simulink library "DQ_SR_LIB_SIM"  (R2019b)
settings: Solver=VariableStepAuto  StartTime=0.0  StopTime=10.0  RelTol=1e-3  EnableMultiTasking=on
undefined symbols (not defined in the file): crossqm, II, II0, magnitude, SATFUNCNAME, X0, XCG0, xi0
(part 1 of 2)
settings Model: Creator=rivolta  LastModifiedBy=AurelianoRivolta
settings DataIOCC: LimitDataPoints=on  ReturnWorkspaceOutputs=off
settings OptimizationCC: LifeSpan=inf
settings DebuggingCC: AllowSymbolicDim=off  SFUnexpectedBacktrackingDiag=warning  SFNoUnconditionalDefaultTransitionDiag=warning  SFExecutionAtInitializationDiag=none  ArithmeticOperatorsInVariantConditions=warning
settings ModelReferenceCC: PropagateSignalLabelsOutOfModel=off
settings SFSimCC: SimUseLocalCustomCode=off  CustomCodeUndefinedFunction=UseInterfaceOnly
settings RTWCC: RTWUseLocalCustomCode=off
settings CodeAppCC: StateflowObjectComments=on
settings GRTTargetCC: TargetLangStandard=C89/C90 (ANSI)
settings ConfigComp: CovMetricSettings=dw  CovHtmlReporting=on  CovSaveCumulativeToWorkspaceVar=on  CovSaveSingleToWorkspaceVar=on  CovExternalEMLEnable=off

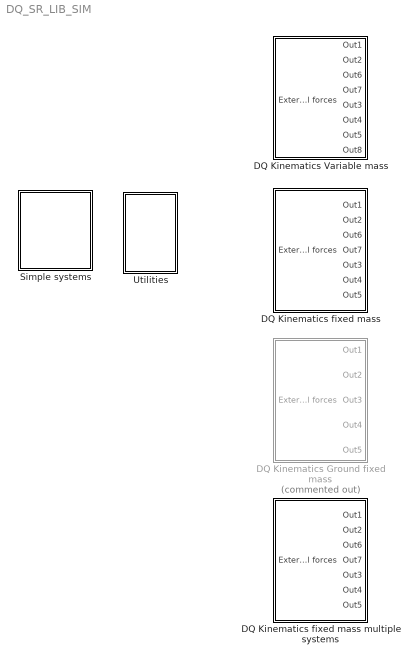
== system DQ_SR_LIB_SIM ==
  DQ Kinematics Ground fixed mass : Subsystem  Commented=on  mask{dynfun=SATFUNCNAME, Gswitch=ECI gravity (F,T), n_bodies=2, n_var0=5, n_ext=7, q_norm_in=[6:9;1:4], II=II, X0=X0, UPPERSAT=Inf, LOWERSAT=-Inf}
      mask prompts: dynfun "System function"; Gswitch "Gravity model"; n_bodies "Number of bodies"; n_var0 "Number of variables"; n_ext "External force size"; q_norm_in "Quaternion indeces"; II "Mass matrix"; X0 "System"; UPPERSAT "Upper Limit"; LOWERSAT "Lower Limit"
      mask init:
      | % check if the incoming function has the correct number of inputs
      | if nargin(dynfun) ~= 9
      |     error('wrong number of inputs, should be: [x,dx,xcg,vcg,time,II,ext_forces,xi]')
      | end
      | 
      | % number of state variables as from input
      | n_var0=length(X0)/2;
      | 
      | % number of bodies from mass conditions
      | n_bodies=size(II,2);
      | 
      | % convert function to be used for trials
      | trialf=str2func(dynfun);
      | gfun=str2func('NO_gravity');
      | 
      | % supposed length of external forces vector
      | n_ext=1;
      | 
      | % check variables
      | CKH=true;
      | iter = 0;
      | line_err=1e5;
      | xi0=0;
      | 
      | while CKH && iter<100
      | 
      |     try 
      |         trialf(ones(n_var0,1),ones(n_var0,1),ones(3,1),ones(3,1),0,II,ones(n_ext,1),xi0,gfun);
      |         CKH=false;
      |     catch M
      |         % catch error line
      |         G=M.stack.line;
      |         % check if the error is after previous line
      |         if (G <= line_err)
      |             n_ext=n_ext+1;
      |         end
      |         % adjourne line error
      |         line_err=G;
      |     end
      |     iter = iter +1;
      |     
      | end
      | 
      | % check if something went wrong. unlikely to have 100 input vector, to be
      | % fixed in later versions
      | if iter >100
      |     warning('likely to have inputs dimension incompatibility')
      | end
      | 
      | % check if I-O dimensions are consistent
      | sys=trialf(X0(n_var0+1:end),X0(1:n_var0),[],[],0,II,ones(n_ext,1),1,gfun);
      | 
      | if sys.n_bodies ~= n_bodies
      |     error('body number inconsistent')
      | end
      | 
      | if sys.nvar ~= n_var0
      |     error ('variable number inconsistent')
      | end
      | 
      | % convert to supply the function name to Mfunction
      | sys_gen_fun_NAME=uint8(dynfun);
      | 
      | % gravity function translation for Mfunction input
      | gravity_fun_NAME = select_gravity_model(Gswitch);
      | 
      | % state and its derivative size
      | n_var=2*n_var0;
      | 
      | % number of variable mass states
      | n_massvar=size(xi0);
      mask Help:
      | % Author: Aureliano Rivolta
      | % e-mail: aureliano.rivolta@polimi.it
      | % year: 2016
      | % private use only
      mask TypeOptions Gswitch: No gravity | Ground gravity (-z) | ECI gravity force | ECI gravity (F,T)
      mask DialogControl Container4 Prompt: System parameters
      mask DialogControl Container5 Prompt: Phisical parameters
      mask DialogControl Control3 Prompt: Initial conditions
      mask DialogControl Container3 Prompt: State Saturation
      mask DialogControl Control2 Prompt: Saturation limits for the system states. If no limits, then put Inf.
      mask Display:
      | port_label('input',1,'f_{ext}','interpreter','tex');
      | port_label('output',1,'v','interpreter','tex');
      | port_label('output',2,'x','interpreter','tex');
      | port_label('output',3,'a','interpreter','tex');
      | port_label('output',4,'da','interpreter','tex');
      | port_label('output',5,'dda','interpreter','tex');
      | fprintf('Ground\nfixed\nmass\nELIMINATO')
  DQ Kinematics Variable mass : Subsystem  mask{dynfun=SATFUNCNAME, Gswitch=No gravity, n_bodies=1, n_var0=4, n_ext=6, q_norm_in=[1:4]', NORMONOFF=on, II=II, xi0=xi0, X0=X0, XCG0=XCG0, UPPERSAT=Inf, LOWERSAT=-Inf}
      mask prompts: dynfun "System function"; Gswitch "Gravity model"; n_bodies "Number of bodies"; n_var0 "Number of variables"; n_ext "External force size"; q_norm_in "Quaternion indeces"; NORMONOFF "Normalize quaternions"; II "Mass matrix"; xi0 "Variable mass IC"; X0 "System"; XCG0 "Center of Mass"; UPPERSAT "Upper Limit"; LOWERSAT "Lower Limit"
      mask init:
      | % check if the incoming function has the correct number of inputs
      | if nargin(dynfun) ~= 9
      |     error('wrong number of inputs, should be: [x,dx,xcg,vcg,time,II,ext_forces,xi,gravity_fun]')
      | end
      | 
      | % number of state variables as from input
      | n_var0=length(X0)/2;
      | 
      | % number of bodies from mass conditions
      | n_bodies=size(II,2);
      | 
      | % convert function to be used for trials
      | trialf=str2func(dynfun);
      | gfun=str2func('NO_gravity');
      | 
      | % supposed length of external forces vector
      | n_ext=1;
      | 
      | % check variables
      | CKH=true;
      | iter = 0;
      | line_err=1e5;
      | 
      | while CKH && iter<100
      | 
      |     try 
      |         trialf(ones(n_var0,1),ones(n_var0,1),ones(3,1),ones(3,1),0,II,ones(n_ext,1),xi0,gfun);
      |         CKH=false;
      |     catch M
      |         % catch error line
      |         G=M.stack.line;
      |         % check if the error is after previous line
      |         if (G <= line_err)
      |             n_ext=n_ext+1;
      |         end
      |         % adjourne line error
      |         line_err=G;
      |     end
      |     iter = iter +1;
      |     
      | end
      | 
      | % check if something went wrong. unlikely to have 100 input vector, to be
      | % fixed in later versions
      | if iter >100
      |     warning('likely to have inputs dimension incompatibility')
      | end
      | 
      | % check if I-O dimensions are consistent
      | sys=trialf(X0(n_var0+1:end),X0(1:n_var0),XCG0(4:end),XCG0(1:3),0,II,ones(n_ext,1),xi0,gfun);
      | 
      | if sys.n_bodies ~= n_bodies
      |     error('body number inconsistent')
      | end
      | 
      | if sys.nvar ~= n_var0
      |     error ('variable number inconsistent')
      | end
      | 
      | % convert to supply the function name to Mfunction
      | sys_gen_fun_NAME=uint8(dynfun);
      | 
      | % gravity function translation for Mfunction input
      | gravity_fun_NAME = select_gravity_model(Gswitch);
      | 
      | % state and its derivative size
      | n_var=2*n_var0;
      | 
      | % number of variable mass states
      | n_massvar=size(xi0);
      mask Help:
      | % Author: Aureliano Rivolta
      | % e-mail: aureliano.rivolta@polimi.it
      | % year: 2016
      | % private use only
      mask TypeOptions Gswitch: No gravity | Ground gravity (-z) | ECI gravity force | ECI gravity (F,T) | CW linearized
      mask DialogControl Container4 Prompt: System parameters
      mask DialogControl Control5 Prompt: Edit
      mask DialogControl Control5 Callback:
      | fun2edit = eval(get_param(gcb,'dynfun'));
      | 
      | edit(fun2edit)
      mask DialogControl Control6 Prompt: New
      mask DialogControl Control6 Callback:
      | directory_string = get_DQ_folder;
      | 
      | copyfile([directory_string,'\simulink_blocks\onesat_S.m'],'template.m')
      | 
      | edit template
      mask DialogControl Container5 Prompt: Phisical parameters
      mask DialogControl Control3 Prompt: Initial conditions
      mask DialogControl Container3 Prompt: State Saturation
      mask DialogControl Control2 Prompt: Saturation limits for the system states. If no limits, then put Inf.
      mask Display:
      | port_label('input',1,'f_{ext}','interpreter','tex');
      | port_label('output',1,'v','interpreter','tex');
      | port_label('output',2,'x','interpreter','tex');
      | port_label('output',3,'v_{cg}','interpreter','tex');
      | port_label('output',4,'x_{cg}','interpreter','tex');
      | port_label('output',5,'a','interpreter','tex');
      | port_label('output',6,'da','interpreter','tex');
      | port_label('output',7,'dda','interpreter','tex');
      | port_label('output',8,'\xi','interpreter','tex');
      | fprintf('variable\nmass')
  DQ Kinematics fixed mass : Subsystem  mask{dynfun=SATFUNCNAME, Gswitch=No gravity, n_bodies=2, n_var0=5, n_ext=7, q_norm_in=[1:4]', NORMONOFF=on, II=II0, X0=X0, XCG0=XCG0, UPPERSAT=Inf, LOWERSAT=-Inf}
      mask prompts: dynfun "System function"; Gswitch "Gravity model:"; n_bodies "Number of bodies"; n_var0 "Number of variables"; n_ext "External force size"; q_norm_in "Quaternion indeces"; NORMONOFF "Normalize quaternion"; II "Mass matrix"; X0 "System"; XCG0 "Center of Mass"; UPPERSAT "Upper Limit"; LOWERSAT "Lower Limit"
      mask init:
      | % check if the incoming function has the correct number of inputs
      | if nargin(dynfun) ~= 9
      |     error('wrong number of inputs, should be: [x,dx,xcg,vcg,time,II,ext_forces,xi]')
      | end
      | 
      | % number of state variables as from input
      | n_var0=length(X0)/2;
      | 
      | % number of bodies from mass conditions
      | n_bodies=size(II,2);
      | 
      | % convert function to be used for trials
      | trialf=str2func(dynfun);
      | gfun=str2func('NO_gravity');
      | 
      | % supposed length of external forces vector
      | n_ext=1;
      | 
      | % check variables
      | CKH=true;
      | iter = 0;
      | line_err=1e5;
      | xi0=0;
      | 
      | 
      | while CKH && iter<100
      | 
      |     try 
      |         trialf(ones(n_var0,1),ones(n_var0,1),ones(3,1),ones(3,1),0,II,ones(n_ext,1),xi0,gfun);
      |         CKH=false;
      |     catch M
      |         % catch error line
      |         G=M.stack.line;
      |         % check if the error is after previous line
      |         if (G <= line_err)
      |             n_ext=n_ext+1;
      |         end
      |         % adjourne line error
      |         line_err=G;
      |     end
      |     iter = iter +1;
      |     
      | end
      | 
      | % check if something went wrong. unlikely to have 100 input vector, to be
      | % fixed in later versions
      | if iter >100
      |     warning('likely to have inputs dimension incompatibility')
      | end
      | 
      | % check if I-O dimensions are consistent
      | sys=trialf(X0(n_var0+1:end),X0(1:n_var0),XCG0(4:end),XCG0(1:3),0,II,ones(n_ext,1),1,gfun);
      | 
      | if sys.n_bodies ~= n_bodies
      |     error('body number inconsistent')
      | end
      | 
      | if sys.nvar ~= n_var0
      |     error ('variable number inconsistent')
      | end
      | 
      | % convert to supply the function name to Mfunction
      | sys_gen_fun_NAME=uint8(dynfun);
      | 
      | % gravity function translation for Mfunction input
      | gravity_fun_NAME = select_gravity_model(Gswitch);
      | 
      | % state and its derivative size
      | n_var=2*n_var0;
      | 
      | % number of variable mass states
      | n_massvar=size(xi0);
      mask Help:
      | % Author: Aureliano Rivolta
      | % e-mail: aureliano.rivolta@polimi.it
      | % year: 2016
      | % private use only
      mask TypeOptions Gswitch: No gravity | Ground gravity (-z) | ECI gravity force | ECI gravity (F,T) | CW linearized model
      mask DialogControl Container4 Prompt: System parameters
      mask DialogControl Control5 Prompt: Edit
      mask DialogControl Control5 Callback:
      | fun2edit = eval(get_param(gcb,'dynfun'));
      | 
      | edit(fun2edit);
      mask DialogControl Control6 Prompt: New
      mask DialogControl Control6 Callback: get_DQSR_template
      mask DialogControl Container5 Prompt: Phisical parameters
      mask DialogControl Control3 Prompt: Initial conditions
      mask DialogControl Container3 Prompt: State Saturation
      mask DialogControl Control2 Prompt: Saturation limits for the system states. If no limits, then put Inf.
      mask Display:
      | port_label('input',1,'f_{ext}','interpreter','tex');
      | port_label('output',1,'v','interpreter','tex');
      | port_label('output',2,'x','interpreter','tex');
      | port_label('output',3,'v_{cg}','interpreter','tex');
      | port_label('output',4,'x_{cg}','interpreter','tex');
      | port_label('output',5,'a','interpreter','tex');
      | port_label('output',6,'da','interpreter','tex');
      | port_label('output',7,'dda','interpreter','tex');
      | fprintf('fixed\nmass')
  DQ Kinematics fixed mass multiple systems : Subsystem  mask{dynfun=SATFUNCNAME, Gswitch=No gravity, n_bodies=2, n_var0=5, n_ext=7, q_norm_in=[1:4;5:8]', NORMONOFF=on, II=II0, X0=X0, XCG0=XCG0, UPPERSAT=Inf, LOWERSAT=-Inf}
      mask prompts: dynfun "System function"; Gswitch "Gravity model"; n_bodies "Number of bodies"; n_var0 "Number of variables"; n_ext "External force size"; q_norm_in "Quaternion indeces"; NORMONOFF "Normalize quaternion"; II "Mass matrix"; X0 "System"; XCG0 "Center of Mass"; UPPERSAT "Upper Limit"; LOWERSAT "Lower Limit"
      mask init:
      | % check if the incoming function has the correct number of inputs
      | if nargin(dynfun) ~= 9
      |     error('wrong number of inputs, should be: [x,dx,xcg,vcg,time,II,ext_forces,xi]')
      | end
      | 
      | % number of state variables as from input
      | n_var0=length(X0)/2;
      | 
      | % number of bodies from mass conditions
      | n_bodies=size(II,2);
      | 
      | % convert function to be used for trials
      | trialf=str2func(dynfun);
      | gfun=str2func('NO_gravity');
      | 
      | % supposed length of external forces vector
      | n_ext=1;
      | 
      | % check variables
      | CKH=true;
      | iter = 0;
      | line_err=1e5;
      | xi0=0;
      | 
      | while CKH && iter<100
      | 
      |     try 
      |         SSS=trialf(X0(n_var0+1:end),X0(1:n_var0),XCG0(4:6,:),XCG0(1:3,:),0,II,ones(n_ext,1),xi0,gfun);
      |         CKH=false;
      | %         SSS
      |     catch M
      |         % catch error line
      |         G=M.stack.line;
      |         % check if the error is after previous line
      |         if (G <= line_err)
      |             n_ext=n_ext+1;
      |         end
      |         % adjourne line error
      |         line_err=G;
      |     end
      |     iter = iter +1;
      |     
      | end
      | 
      | % check if something went wrong. unlikely to have 100 input vector, to be
      | % fixed in later versions
      | if iter >100
      |     warning('likely to have inputs dimension incompatibility')
      | end
      | 
      | % check if I-O dimensions are consistent
      | systems=trialf(X0(n_var0+1:end),X0(1:n_var0),XCG0(4:6,:),XCG0(1:3,:),0,II,ones(n_ext,1),1,gfun);
      | ns=length(systems);
      | 
      | %check bodies and variable numbers
      | [nb,nv]=deal(zeros(1,ns));
      | for i=1:ns
      |     nb(i)=systems(i).n_bodies;
      |     nv(i)=systems(i).nvar;
      | end
      | 
      | if sum(nb) ~= n_bodies
      |     error('body number inconsistent')
      | end
      | 
      | if sum(nv) ~= n_var0
      |     error ('variable number inconsistent')
      | end
      | 
      | % convert to supply the function name to Mfunction
      | sys_gen_fun_NAME=uint8(dynfun);
      | 
      | % gravity function translation for Mfunction input
      | gravity_fun_NAME = select_gravity_model(Gswitch);
      | 
      | % state and its derivative size
      | n_var=2*n_var0;
      | 
      | % number of variable mass states
      | n_massvar=size(xi0);
      | 
      | % initialize the contact memory matrix
      | nc=sum(sum(nb'*nb-diag(diag(nb'*nb))))/2;
      | vref0=zeros(6,nc);
      | 
      | % initialize the contact table
      | CONTACTABLE0=[];
      | 
      | for i=1:ns-1
      |     for k=1:nb(i)
      |         for j=i+1:ns
      |             for l=1:nb(j)
      |                 CONTACTABLE0=[CONTACTABLE0;[i,k,j,l]];
      |             end
      |         end
      |     end
      | end
      | 
      | % disable warnings. not the best options but in many cases there will be
      | % warnings for some parallel faces in the contact determination. In the
      | % future cases then 
      | warning off
      mask Help:
      | % Author: Aureliano Rivolta
      | % e-mail: aureliano.rivolta@polimi.it
      | % year: 2016
      | % private use only
      mask TypeOptions Gswitch: No gravity | Ground gravity (-z) | ECI gravity force | ECI gravity (F,T) | CW linearized model
      mask DialogControl Container4 Prompt: System parameters
      mask DialogControl Control5 Prompt: Edit
      mask DialogControl Control5 Callback:
      | fun2edit = eval(get_param(gcb,'dynfun'));
      | 
      | edit(fun2edit)
      mask DialogControl Control6 Prompt: New
      mask DialogControl Control6 Callback: get_DQSR_template
      mask DialogControl Container5 Prompt: Phisical parameters
      mask DialogControl Control3 Prompt: Initial conditions
      mask DialogControl Container3 Prompt: State Saturation
      mask DialogControl Control2 Prompt: Saturation limits for the system states. If no limits, then put Inf.
      mask Display:
      | port_label('input',1,'f_{ext}','interpreter','tex');
      | port_label('output',1,'v','interpreter','tex');
      | port_label('output',2,'x','interpreter','tex');
      | port_label('output',3,'v_{cg}','interpreter','tex');
      | port_label('output',4,'x_{cg}','interpreter','tex');
      | port_label('output',5,'a','interpreter','tex');
      | port_label('output',6,'da','interpreter','tex');
      | port_label('output',7,'dda','interpreter','tex');
      | fprintf('fixed\nmass\nsystems')
  Simple systems : Subsystem
      settings: OpenFcn=SAMPLE_systems
  Utilities : Subsystem

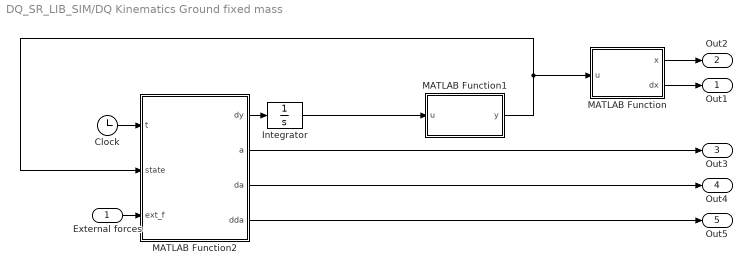
== system DQ_SR_LIB_SIM/DQ Kinematics Ground fixed mass ==
  External forces : Inport
  Clock : Clock
  Integrator : Integrator  InitialCondition=X0  LimitOutput=on  UpperSaturationLimit=UPPERSAT  LowerSaturationLimit=LOWERSAT
  MATLAB Function : MATLAB Function  TreatAsAtomicUnit=on  mask{n_states=n_var}
      mask prompts: n_states "Number of states"
  MATLAB Function1 : MATLAB Function  TreatAsAtomicUnit=on  mask{qindex=q_norm_in}
      mask prompts: qindex "Quaternion index"
      mask init:
      | index=qindex(1,:);
      | index2=qindex(2,:);
  MATLAB Function2 : MATLAB Function  TreatAsAtomicUnit=on
  Out1 : Outport
  Out2 : Outport  Port=2
  Out3 : Outport  Port=3
  Out4 : Outport  Port=4
  Out5 : Outport  Port=5
  wires:
  Clock/1 -> MATLAB Function2/1(t)
  MATLAB Function2/4(dda) -> Out5/1
  MATLAB Function/1(x) -> Out2/1
  MATLAB Function/2(dx) -> Out1/1
  MATLAB Function2/1(dy) -> Integrator/1
  MATLAB Function2/2(a) -> Out3/1
  MATLAB Function2/3(da) -> Out4/1
  External forces/1 -> MATLAB Function2/3(ext_f)
  Integrator/1 -> MATLAB Function1/1(u)
  MATLAB Function1/1(y) -> MATLAB Function/1(u), MATLAB Function2/2(state)

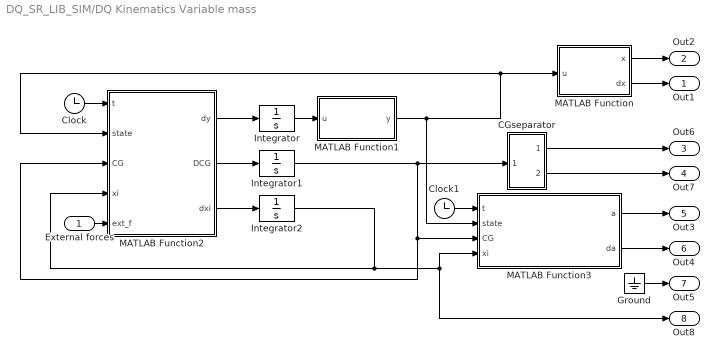
== system DQ_SR_LIB_SIM/DQ Kinematics Variable mass ==
  External forces : Inport
  CGseparator : Subsystem
      mask Display:
      | port_label('input',1,'CG')
      | port_label('output',1,'v_{cg}','interpreter','tex')
      | port_label('output',2,'x_{cg}','interpreter','tex')
  Clock : Clock
  Clock1 : Clock
  Ground : Ground
  Integrator : Integrator  InitialCondition=X0  LimitOutput=on  UpperSaturationLimit=UPPERSAT  LowerSaturationLimit=LOWERSAT
  Integrator1 : Integrator  InitialCondition=XCG0
  Integrator2 : Integrator  InitialCondition=xi0  LimitOutput=on  UpperSaturationLimit=1  LowerSaturationLimit=0
  MATLAB Function : MATLAB Function  TreatAsAtomicUnit=on  mask{n_states=n_var}
      mask prompts: n_states "Number of states"
  MATLAB Function1 : MATLAB Function  TreatAsAtomicUnit=on  mask{qindex=q_norm_in}
      mask prompts: qindex "Quaternion index"
  MATLAB Function2 : MATLAB Function  TreatAsAtomicUnit=on
  MATLAB Function3 : MATLAB Function  TreatAsAtomicUnit=on
  Out1 : Outport
  Out2 : Outport  Port=2
  Out6 : Outport  Port=3
  Out7 : Outport  Port=4
  Out3 : Outport  Port=5
  Out4 : Outport  Port=6
  Out5 : Outport  Port=7
  Out8 : Outport  Port=8
  wires:
  Integrator/1 -> MATLAB Function1/1(u)
  Integrator2/1 -> Out8/1, MATLAB Function3/4(xi), MATLAB Function2/4(xi)
  CGseparator/2(Out3) -> Out7/1
  External forces/1 -> MATLAB Function2/5(ext_f)
  MATLAB Function/2(dx) -> Out1/1
  MATLAB Function/1(x) -> Out2/1
  MATLAB Function2/2(DCG) -> Integrator1/1
  Clock/1 -> MATLAB Function2/1(t)
  CGseparator/1(Out1) -> Out6/1
  MATLAB Function2/3(dxi) -> Integrator2/1
  MATLAB Function1/1(y) -> MATLAB Function3/2(state), MATLAB Function2/2(state), MATLAB Function/1(u)
  MATLAB Function2/1(dy) -> Integrator/1
  Integrator1/1 -> CGseparator/1(In1), MATLAB Function2/3(CG), MATLAB Function3/3(CG)
  Clock1/1 -> MATLAB Function3/1(t)
  MATLAB Function3/1(a) -> Out3/1
  MATLAB Function3/2(da) -> Out4/1
  Ground/1 -> Out5/1

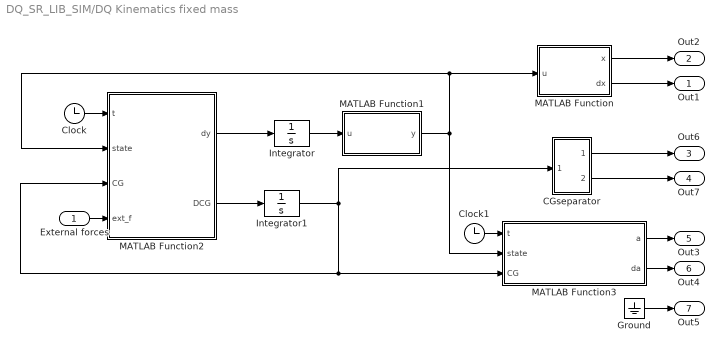
== system DQ_SR_LIB_SIM/DQ Kinematics fixed mass ==
  External forces : Inport
  CGseparator : Subsystem
      mask Display:
      | port_label('input',1,'CG')
      | port_label('output',1,'v_{cg}','interpreter','tex')
      | port_label('output',2,'x_{cg}','interpreter','tex')
  Clock : Clock
  Clock1 : Clock
  Ground : Ground
  Integrator : Integrator  InitialCondition=X0  LimitOutput=on  UpperSaturationLimit=UPPERSAT  LowerSaturationLimit=LOWERSAT
  Integrator1 : Integrator  InitialCondition=XCG0
  MATLAB Function : MATLAB Function  TreatAsAtomicUnit=on  mask{n_states=n_var}
      mask prompts: n_states "Number of states"
  MATLAB Function1 : MATLAB Function  TreatAsAtomicUnit=on  mask{qindex=q_norm_in}
      mask prompts: qindex "Quaternion index"
  MATLAB Function2 : MATLAB Function  TreatAsAtomicUnit=on
  MATLAB Function3 : MATLAB Function  TreatAsAtomicUnit=on
  Out1 : Outport
  Out2 : Outport  Port=2
  Out6 : Outport  Port=3
  Out7 : Outport  Port=4
  Out3 : Outport  Port=5
  Out4 : Outport  Port=6
  Out5 : Outport  Port=7
  wires:
  MATLAB Function1/1(y) -> MATLAB Function2/2(state), MATLAB Function/1(u), MATLAB Function3/2(state)
  CGseparator/2(Out3) -> Out7/1
  Integrator/1 -> MATLAB Function1/1(u)
  External forces/1 -> MATLAB Function2/4(ext_f)
  MATLAB Function2/1(dy) -> Integrator/1
  MATLAB Function/2(dx) -> Out1/1
  MATLAB Function/1(x) -> Out2/1
  MATLAB Function2/2(DCG) -> Integrator1/1
  Integrator1/1 -> CGseparator/1(In1), MATLAB Function3/3(CG), MATLAB Function2/3(CG)
  Clock/1 -> MATLAB Function2/1(t)
  CGseparator/1(Out1) -> Out6/1
  Clock1/1 -> MATLAB Function3/1(t)
  MATLAB Function3/1(a) -> Out3/1
  MATLAB Function3/2(da) -> Out4/1
  Ground/1 -> Out5/1

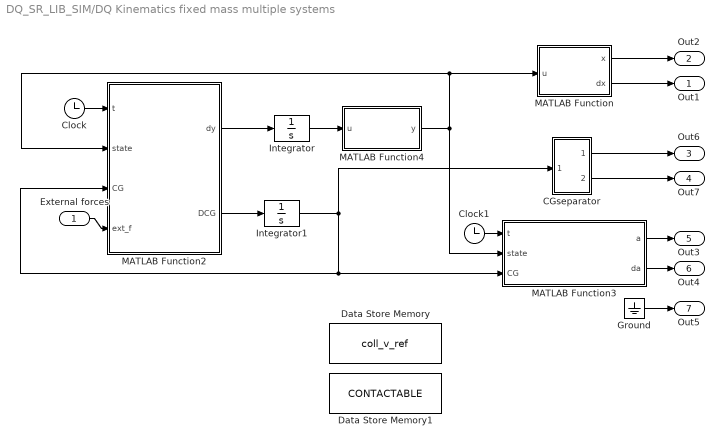
== system DQ_SR_LIB_SIM/DQ Kinematics fixed mass multiple systems ==
  External forces : Inport
  CGseparator : Subsystem
      mask Display:
      | port_label('input',1,'CG')
      | port_label('output',1,'v_{cg}','interpreter','tex')
      | port_label('output',2,'x_{cg}','interpreter','tex')
  Clock : Clock
  Clock1 : Clock
  Data Store Memory : DataStoreMemory  DataStoreName=coll_v_ref  ReadBeforeWriteMsg=warning  WriteAfterWriteMsg=warning  WriteAfterReadMsg=warning  InitialValue=vref0  VectorParams1D=off  ShowAdditionalParam=off  OutDataTypeStr=double  Dimensions=[6,nc]
  Data Store Memory1 : DataStoreMemory  DataStoreName=CONTACTABLE  ReadBeforeWriteMsg=warning  WriteAfterWriteMsg=warning  WriteAfterReadMsg=warning  InitialValue=CONTACTABLE0  VectorParams1D=off  ShowAdditionalParam=off  OutDataTypeStr=double  Dimensions=[nc,4]
  Ground : Ground
  Integrator : Integrator  InitialCondition=X0  LimitOutput=on  UpperSaturationLimit=UPPERSAT  LowerSaturationLimit=LOWERSAT
  Integrator1 : Integrator  InitialCondition=XCG0
  MATLAB Function : MATLAB Function  TreatAsAtomicUnit=on  mask{n_states=n_var}
      mask prompts: n_states "Number of states"
  MATLAB Function2 : MATLAB Function  TreatAsAtomicUnit=on
  MATLAB Function3 : MATLAB Function  TreatAsAtomicUnit=on
  MATLAB Function4 : MATLAB Function  TreatAsAtomicUnit=on  mask{qindex=q_norm_in}
      mask prompts: qindex "Quaternion index"
  Out1 : Outport
  Out2 : Outport  Port=2
  Out6 : Outport  Port=3
  Out7 : Outport  Port=4
  Out3 : Outport  Port=5
  Out4 : Outport  Port=6
  Out5 : Outport  Port=7
  wires:
  MATLAB Function2/2(DCG) -> Integrator1/1
  Ground/1 -> Out5/1
  MATLAB Function3/2(da) -> Out4/1
  MATLAB Function3/1(a) -> Out3/1
  Clock1/1 -> MATLAB Function3/1(t)
  CGseparator/1(Out1) -> Out6/1
  Clock/1 -> MATLAB Function2/1(t)
  Integrator1/1 -> MATLAB Function2/3(CG), MATLAB Function3/3(CG), CGseparator/1(In1)
  MATLAB Function/1(x) -> Out2/1
  MATLAB Function/2(dx) -> Out1/1
  MATLAB Function2/1(dy) -> Integrator/1
  External forces/1 -> MATLAB Function2/4(ext_f)
  Integrator/1 -> MATLAB Function4/1(u)
  CGseparator/2(Out3) -> Out7/1
  MATLAB Function4/1(y) -> MATLAB Function/1(u), MATLAB Function2/2(state), MATLAB Function3/2(state)

== system DQ_SR_LIB_SIM/Simple systems ==

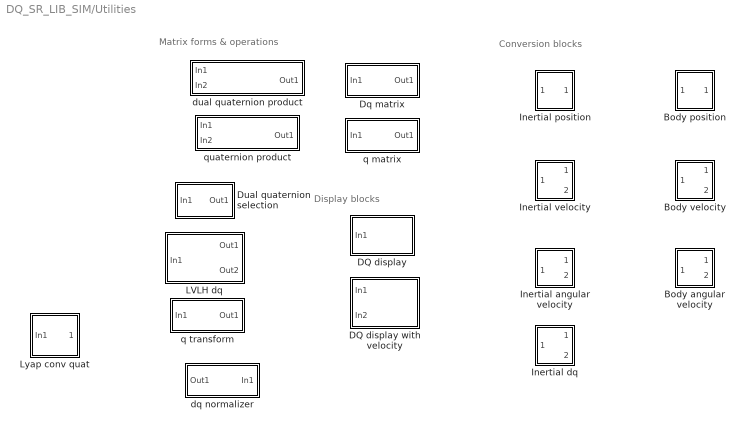
== system DQ_SR_LIB_SIM/Utilities ==
  note: Matrix forms & operations
  note: Conversion blocks
  note: Display blocks
  Body angular velocity : Subsystem
      mask help: Body relative angular velocity
      mask Display:
      | port_label('input',1,'q')
      | port_label('input',2,'dq','interpreter','tex')
      | port_label('output',1,'\omega_b','interpreter','tex')
  Body position : Subsystem
      mask help: Body relative position
      mask Display:
      | port_label('input',1,'a')
      | 
      | port_label('output',1,'d_b','interpreter','tex')
  Body velocity : Subsystem
      mask help: Body relative position
      mask Display:
      | port_label('input',1,'a')
      | port_label('input',2,'da')
      | 
      | port_label('output',1,'v_b','interpreter','tex')
  DQ display : Subsystem  mask{ST=10, NFIG=1}
      mask prompts: ST "Sample time"; NFIG "Figure id"
      mask init:
      | figure(NFIG)
      | % close(NFIG)
      | % figure(NFIG)
      | % subplot(1,2,1)
      | % view(30,30)
      mask DialogControl Control2 Prompt: Reset
      mask DialogControl Control2 Callback: close(eval(get_param(gcb,'NFIG')));
      mask Display:
      | fprintf('DQ\nDisplay')
      | port_label('input',1,'a')
  DQ display with velocity : Subsystem  mask{ST=1, NFIG=1}
      mask prompts: ST "Sample time"; NFIG "Figure id"
      mask init:
      | figure(NFIG)
      | % close(NFIG)
      | % figure(NFIG)
      | % subplot(1,2,1)
      | % view(30,30)
      mask Display:
      | fprintf('DQ\nDisplay\nVelocity')
      | port_label('input',1,'a')
      | port_label('input',2,'da')
  Dq matrix : Subsystem  mask{dqfun=dq product -}
      mask prompts: dqfun "Dq function"
      mask init:
      | switch dqfun
      | %     dq product -
      | %     dq product +
      | %     dq product - transpose
      | %     dq product + transpose
      | %     dq division -
      | %     dq division +
      | %     dq division - transpose
      | %     dq division + transpose
      | %     dq conjugate
      |     case 1
      |         dqfunchar='dqprodm';
      |     case 2
      |         dqfunchar='dqprodp';
      |     case 3
      |         dqfunchar='dqprodmt';
      |     case 4
      |         dqfunchar='dqprodpt';
      |     case 5
      |         dqfunchar='dqdivm';
      |     case 6
      |         dqfunchar='dqdivp';
      |     case 7
      |         dqfunchar='dqdivmt';
      |     case 8
      |         dqfunchar='dqdivpt';
      |     case 9
      |         dqfunchar='dq_conj';
      | end
      | 
      | fun_NAME=uint8(dqfunchar);
      mask TypeOptions dqfun: dq product - | dq product + | dq product - transpose | dq product + transpose | dq division - | dq division + | dq division - transpose | dq division + transpose | conjugate
      mask Display: fprintf(dqfunchar)
  Dual quaternion selection : Subsystem  RequirementInfo="{}  %GIDa_e34a7cc5_2e61_475f_b9f9_c475a4dcd3f7"  mask{x=1:4, y=1}
      mask prompts: x "dq quaternion indeces"; y "body indeces"
      mask Help:
      | % Author: Aureliano Rivolta
      | % e-mail: aureliano.rivolta@polimi.it
      | % year: 2016
      | % private use only
      mask Display: fprintf('DQ\nselection')
  Inertial angular velocity : Subsystem
      mask help: Inertial angular velocity
      mask Display:
      | port_label('input',1,'q')
      | port_label('input',2,'dq','interpreter','tex')
      | port_label('output',1,'\omega_i','interpreter','tex')
  Inertial dq : Subsystem
      mask help: DQ generation from inertial conditions
      mask Display:
      | port_label('output',1,'a')
      | 
      | port_label('input',1,'d_i','interpreter','tex')
      | port_label('input',2,'q','interpreter','tex')
  Inertial position : Subsystem
      mask help: Inertial position
      mask Display:
      | port_label('input',1,'a')
      | 
      | port_label('output',1,'d_i','interpreter','tex')
  Inertial velocity : Subsystem
      mask help: Inertial position
      mask Display:
      | port_label('input',1,'a')
      | port_label('input',2,'da')
      | 
      | port_label('output',1,'v_i','interpreter','tex')
  LVLH dq : Subsystem  mask{mu=3.986*10^5*1e9, d0=(6371+413)*1e3, RAAN=0, i=0, theta=0}
      mask prompts: mu "Gravity parameter [m^3/s^2]"; d0 "Orbit radius [m]"; RAAN "RAAN [rad]"; i "Inclination [rad]"; theta "Initial anomaly [rad]"
      mask init:
      | % angular velocity
      | n = sqrt (mu / (d0^3));
      | 
      | % initial attitude of the lvlh frame
      | q0 = crossqm([sin(i/2);0;0;cos(i/2)])*[0;0;sin(RAAN/2);cos(RAAN/2)];
      mask Display:
      | fprintf('LVLH\ne = 0')
      | port_label('input',1,'t')
      | port_label('output',1,'r')
      | port_label('output',2,'dr')
  Lyap conv quat : Subsystem
      mask Display:
      | port_label('input',1,'q')
      | port_label('output',1,'(1-\epsilon^2)','interpreter','tex')
  dq normalizer : Subsystem
      mask Display: fprintf('DQ normalizer')
  dual quaternion product : Subsystem  mask{ISTRANSPOSE=off, qfun=dq prod -}
      mask prompts: ISTRANSPOSE "Transpose"; qfun "Q function:"
      mask init:
      | switch qfun
      |     case 1
      |         qfunchar='dqprodm';
      |     case 2
      |         qfunchar='dqprodp';
      |     case 3
      |         qfunchar='dqprodmt';
      |     case 4
      |         qfunchar='dqprodpt';
      |     case 5
      |         qfunchar='dqdivm';
      |     case 6
      |         qfunchar='dqdivp';
      |     case 7
      |         qfunchar='dqdivmt';
      |     case 8
      |         qfunchar='dqdivpt';
      | end
      | 
      | fun_NAME=uint8(qfunchar);
      mask TypeOptions qfun: dq prod - | dq prod + | dq prod - T | dq prod + T | dq div - | dq div + | dq div - T | dq div + T
      mask Display:
      | port_label('input',1,'a_1','interpreter','tex')
      | port_label('input',2,'a_2','interpreter','tex')
      | if ISTRANSPOSE
      | fprintf([qfunchar,'(a1)T','*a2'])
      | else
      | fprintf([qfunchar,'(a1)*a2'])
      | end
  q matrix : Subsystem  RequirementInfo="{}  %GIDa_8cae52d0_75ce_45c8_9ca9_047a24feff7a"  mask{qfun=q cross -}
      mask prompts: qfun "Dq function"
      mask init:
      | switch qfun
      |     case 1
      |         qfunchar='crossqm';
      |     case 2
      |         qfunchar='crossqp';
      |     case 3
      |         qfunchar='crossqmt';
      |     case 4
      |         qfunchar='crossqpt';
      |     case 5
      |         qfunchar='q2dcm';
      |     case 6
      |         qfunchar='qconj';
      | end
      | 
      | fun_NAME=uint8(qfunchar);
      mask TypeOptions qfun: q cross - | q cross + | q cross - T | q cross + T | DCM | conjugate
      mask Display: fprintf(qfunchar)
  q transform : Subsystem  mask{qfun=xi --> q}
      mask prompts: qfun "Dq function"
      mask init:
      | switch qfun
      |     case 1
      |         qfunchar='q2minimal';
      |     case 2
      |         qfunchar='minimal2q';
      | end
      | 
      | fun_NAME=uint8(qfunchar);
      mask TypeOptions qfun: q --> xi | xi --> q
      mask Display: fprintf(qfunchar)
  quaternion product : Subsystem  mask{ISTRANSPOSE=off, qfun=DCM}
      mask prompts: ISTRANSPOSE "Transpose"; qfun "Q function:"
      mask init:
      | switch qfun
      |     case 1
      |         qfunchar='crossqm';
      |     case 2
      |         qfunchar='crossqp';
      |     case 3
      |         qfunchar='crossqmt';
      |     case 4
      |         qfunchar='crossqpt';
      |     case 5
      |         qfunchar='q2dcm';
      | end
      | 
      | fun_NAME=uint8(qfunchar);
      mask TypeOptions qfun: q cross - | q cross + | q cross - T | q cross + T | DCM
      mask Display:
      | if qfun == 5
      |     port_label('input',1,'q','interpreter','tex')
      |     port_label('input',2,'v','interpreter','tex')
      | 
      |     if ISTRANSPOSE
      |         fprintf(['R(q1)T','*v'])
      |     else
      |         fprintf(['R(q1)*v'])
      |     end
      | 
      | else
      | 
      |     port_label('input',1,'q_1','interpreter','tex')
      |     port_label('input',2,'q_2','interpreter','tex')
      |     if ISTRANSPOSE
      |         fprintf([qfunchar,'(q1)T','*q2'])
      |     else
      |         fprintf([qfunchar,'(q1)*q2'])
      |     end
      | 
      | end

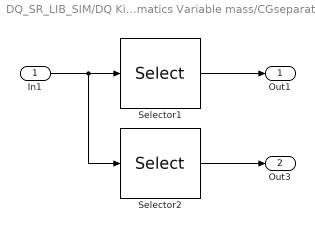
== system DQ_SR_LIB_SIM/DQ Kinematics Variable mass/CGseparator ==
  In1 : Inport
  Selector1 : Selector  InputPortWidth=6  IndexOptions=Index vector (dialog)  Indices=[1:3]  OutputSizes=1
  Selector2 : Selector  InputPortWidth=6  IndexOptions=Index vector (dialog)  Indices=[4:6]  OutputSizes=1
  Out1 : Outport
  Out3 : Outport  Port=2
  wires:
  Selector2/1 -> Out3/1
  Selector1/1 -> Out1/1
  In1/1 -> Selector1/1, Selector2/1

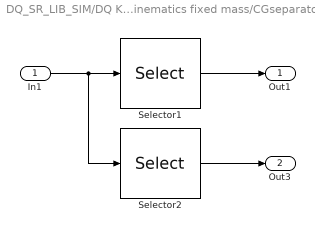
== system DQ_SR_LIB_SIM/DQ Kinematics fixed mass/CGseparator ==
  In1 : Inport
  Selector1 : Selector  InputPortWidth=6  IndexOptions=Index vector (dialog)  Indices=[1:3]  OutputSizes=1
  Selector2 : Selector  InputPortWidth=6  IndexOptions=Index vector (dialog)  Indices=[4:6]  OutputSizes=1
  Out1 : Outport
  Out3 : Outport  Port=2
  wires:
  Selector2/1 -> Out3/1
  Selector1/1 -> Out1/1
  In1/1 -> Selector1/1, Selector2/1

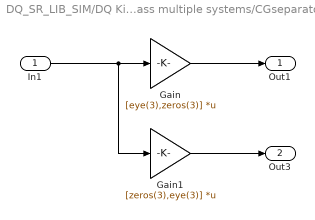
== system DQ_SR_LIB_SIM/DQ Kinematics fixed mass multiple systems/CGseparator ==
  In1 : Inport
  Gain : Gain  Gain=[eye(3),zeros(3)]  Multiplication=Matrix(K*u)
  Gain1 : Gain  Gain=[zeros(3),eye(3)]  Multiplication=Matrix(K*u)
  Out1 : Outport
  Out3 : Outport  Port=2
  wires:
  In1/1 -> Gain/1, Gain1/1
  Gain/1 -> Out1/1
  Gain1/1 -> Out3/1

== system DQ_SR_LIB_SIM/Utilities/Body angular velocity ==
  In1 : Inport
  In2 : Inport  Port=2
  MATLAB Function : MATLAB Function  TreatAsAtomicUnit=on
  Out1 : Outport
  wires:
  In2/1 -> MATLAB Function/2(dq)
  MATLAB Function/1(omega) -> Out1/1
  In1/1 -> MATLAB Function/1(q)

== system DQ_SR_LIB_SIM/Utilities/Body position ==
  In1 : Inport
  MATLAB Function : MATLAB Function  TreatAsAtomicUnit=on
  Out1 : Outport
  wires:
  In1/1 -> MATLAB Function/1(a)
  MATLAB Function/1(d) -> Out1/1

== system DQ_SR_LIB_SIM/Utilities/Body velocity ==
  In1 : Inport
  In2 : Inport  Port=2
  MATLAB Function : MATLAB Function  TreatAsAtomicUnit=on
  Out1 : Outport
  wires:
  In2/1 -> MATLAB Function/2(da)
  In1/1 -> MATLAB Function/1(a)
  MATLAB Function/1(d) -> Out1/1

== system DQ_SR_LIB_SIM/Utilities/DQ display ==
  In1 : Inport
  Level-2 MATLAB S-Function : M-S-Function  FunctionName=DQ_viewer  Parameters=ST,NFIG
  wires:
  In1/1 -> Level-2 MATLAB S-Function/1

== system DQ_SR_LIB_SIM/Utilities/DQ display with velocity ==
  In1 : Inport
  In2 : Inport  Port=2
  Level-2 MATLAB S-Function : M-S-Function  FunctionName=DQ_viewer_vel  Parameters=ST,NFIG
  wires:
  In2/1 -> Level-2 MATLAB S-Function/2
  In1/1 -> Level-2 MATLAB S-Function/1

== system DQ_SR_LIB_SIM/Utilities/Dq matrix ==
  In1 : Inport
  MATLAB Function : MATLAB Function  TreatAsAtomicUnit=on
  Out1 : Outport
  wires:
  In1/1 -> MATLAB Function/1(u)
  MATLAB Function/1(y) -> Out1/1

== system DQ_SR_LIB_SIM/Utilities/Dual quaternion selection ==
  In1 : Inport
  MATLAB Function : MATLAB Function  TreatAsAtomicUnit=on
  Out1 : Outport
  wires:
  MATLAB Function/1(a_xy) -> Out1/1
  In1/1 -> MATLAB Function/1(a)

== system DQ_SR_LIB_SIM/Utilities/Inertial angular velocity ==
  In1 : Inport
  In2 : Inport  Port=2
  MATLAB Function : MATLAB Function  TreatAsAtomicUnit=on
  Out1 : Outport
  wires:
  In1/1 -> MATLAB Function/1(q)
  MATLAB Function/1(omega) -> Out1/1
  In2/1 -> MATLAB Function/2(dq)

== system DQ_SR_LIB_SIM/Utilities/Inertial dq ==
  In1 : Inport
  In2 : Inport  Port=2
  MATLAB Function : MATLAB Function  TreatAsAtomicUnit=on
  Out1 : Outport
  wires:
  In2/1 -> MATLAB Function/2(q)
  MATLAB Function/1(a) -> Out1/1
  In1/1 -> MATLAB Function/1(d)

== system DQ_SR_LIB_SIM/Utilities/Inertial position ==
  In1 : Inport
  MATLAB Function : MATLAB Function  TreatAsAtomicUnit=on
  Out1 : Outport
  wires:
  MATLAB Function/1(d) -> Out1/1
  In1/1 -> MATLAB Function/1(a)

== system DQ_SR_LIB_SIM/Utilities/Inertial velocity ==
  In1 : Inport
  In2 : Inport  Port=2
  MATLAB Function : MATLAB Function  TreatAsAtomicUnit=on
  Out1 : Outport
  wires:
  In2/1 -> MATLAB Function/2(da)
  MATLAB Function/1(d) -> Out1/1
  In1/1 -> MATLAB Function/1(a)

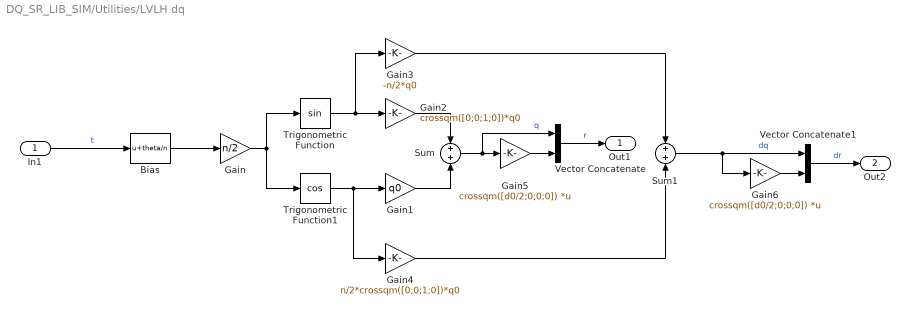
== system DQ_SR_LIB_SIM/Utilities/LVLH dq ==
  In1 : Inport
  Bias : Bias  Bias=theta/n
  Gain : Gain  Gain=n/2
  Gain1 : Gain  Gain=q0
  Gain2 : Gain  Gain=crossqm([0;0;1;0])*q0
  Gain3 : Gain  Gain=-n/2*q0
  Gain4 : Gain  Gain=n/2*crossqm([0;0;1;0])*q0
  Gain5 : Gain  Gain=crossqm([d0/2;0;0;0])  Multiplication=Matrix(K*u)
  Gain6 : Gain  Gain=crossqm([d0/2;0;0;0])  Multiplication=Matrix(K*u)
  Sum : Sum
  Sum1 : Sum
  Trigonometric Function : Trigonometry
  Trigonometric Function1 : Trigonometry  Operator=cos
  Vector Concatenate : Concatenate
  Vector Concatenate1 : Concatenate
  Out1 : Outport
  Out2 : Outport  Port=2
  wires:
  In1/1 -> Bias/1  "t"
  Gain/1 -> Trigonometric Function1/1, Trigonometric Function/1
  Trigonometric Function/1 -> Gain3/1, Gain2/1
  Trigonometric Function1/1 -> Gain4/1, Gain1/1
  Gain2/1 -> Sum/1
  Gain1/1 -> Sum/2
  Sum/1 -> Vector Concatenate/1, Gain5/1  "q"
  Gain3/1 -> Sum1/1
  Gain4/1 -> Sum1/2
  Sum1/1 -> Vector Concatenate1/1, Gain6/1  "dq"
  Gain5/1 -> Vector Concatenate/2
  Gain6/1 -> Vector Concatenate1/2
  Vector Concatenate/1 -> Out1/1  "r"
  Vector Concatenate1/1 -> Out2/1  "dr"
  Bias/1 -> Gain/1

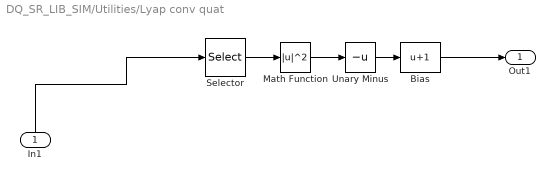
== system DQ_SR_LIB_SIM/Utilities/Lyap conv quat ==
  In1 : Inport
  Bias : Bias  Bias=1
  Math Function : Math  Operator=magnitude^2  SaturateOnIntegerOverflow=on
  Selector : Selector  InputPortWidth=4  IndexOptions=Index vector (dialog)  Indices=[4]  OutputSizes=1
  Unary Minus : UnaryMinus
  Out1 : Outport
  wires:
  Unary Minus/1 -> Bias/1
  Selector/1 -> Math Function/1
  In1/1 -> Selector/1
  Bias/1 -> Out1/1
  Math Function/1 -> Unary Minus/1

== system DQ_SR_LIB_SIM/Utilities/dq normalizer ==
  In1 : Inport
  MATLAB Function : MATLAB Function  TreatAsAtomicUnit=on
  Out1 : Outport
  wires:
  MATLAB Function/1(y) -> Out1/1
  In1/1 -> MATLAB Function/1(u)

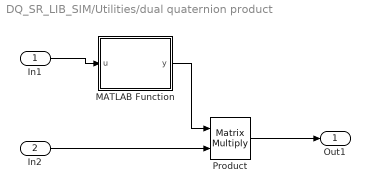
== system DQ_SR_LIB_SIM/Utilities/dual quaternion product ==
  In1 : Inport
  In2 : Inport  Port=2
  MATLAB Function : MATLAB Function  TreatAsAtomicUnit=on
  Product : Product  Multiplication=Matrix(*)
  Out1 : Outport
  wires:
  Product/1 -> Out1/1
  In2/1 -> Product/2
  MATLAB Function/1(y) -> Product/1
  In1/1 -> MATLAB Function/1(u)

== system DQ_SR_LIB_SIM/Utilities/q matrix ==
  In1 : Inport
  MATLAB Function : MATLAB Function  TreatAsAtomicUnit=on
  Out1 : Outport
  wires:
  MATLAB Function/1(y) -> Out1/1
  In1/1 -> MATLAB Function/1(u)

== system DQ_SR_LIB_SIM/Utilities/q transform ==
  In1 : Inport
  MATLAB Function : MATLAB Function  TreatAsAtomicUnit=on
  Out1 : Outport
  wires:
  MATLAB Function/1(y) -> Out1/1
  In1/1 -> MATLAB Function/1(u)

== system DQ_SR_LIB_SIM/Utilities/quaternion product ==
  In1 : Inport
  In2 : Inport  Port=2
  MATLAB Function : MATLAB Function  TreatAsAtomicUnit=on
  Product : Product  Multiplication=Matrix(*)
  Out1 : Outport
  wires:
  Product/1 -> Out1/1
  In2/1 -> Product/2
  MATLAB Function/1(y) -> Product/1
  In1/1 -> MATLAB Function/1(u)

== matlab function DQ_SR_LIB_SIM/DQ Kinematics Variable mass/MATLAB Function ==
  data: u input; x output; dx output; n_states parameter
function [x,dx] = fcn(u,n_states)
%#codegen

% velocity and position of cg included

dx = u (1:(n_states/2),1);

x = u ((n_states/2+1):n_states,1);

== matlab function DQ_SR_LIB_SIM/DQ Kinematics fixed mass/MATLAB Function ==
  data: u input; x output; dx output; n_states parameter
function [x,dx] = fcn(u,n_states)
%#codegen

% velocity and position of cg included

dx = u (1:(n_states/2),1);

x = u ((n_states/2+1):n_states,1);

== matlab function DQ_SR_LIB_SIM/DQ Kinematics Variable mass/MATLAB Function1 ==
  data: u input; y output; qindex parameter; NORMONOFF parameter
function y = quatnormalize(u,qindex,NORMONOFF)
%#codegen

y = u;

if NORMONOFF

    n_state=length(u)/2; % number of states
    
    qindex2=qindex+(n_state); %get quaternion index
    
    
    for i=1:size(qindex,2)
    
        % extract quaternion and its derivative
        q=u(qindex2(:,i));
        dq=u(qindex(:,i));
        
        % quat norm
        q=q./norm(q);
        
        % dquat norm
        Q=crossqm(q);
        omega2=Q'*dq;omega2(4)=0;
        dq=Q*omega2;
    
        y(qindex2(:,i))=q;
        y(qindex(:,i))=dq;
        
    end
    

end

== matlab function DQ_SR_LIB_SIM/DQ Kinematics fixed mass/MATLAB Function1 ==
  data: u input; y output; qindex parameter; NORMONOFF parameter
function y = quatnormalize(u,qindex,NORMONOFF)
%#codegen

y = u;

if NORMONOFF

    n_state=length(u)/2; % number of states
    
    qindex2=qindex+(n_state); %get quaternion index
    
    
    for i=1:size(qindex,2)
    
        % extract quaternion and its derivative
        q=u(qindex2(:,i));
        dq=u(qindex(:,i));
        
        % quat norm
        q=q./norm(q);
        
        % dquat norm
        Q=crossqm(q);
        omega2=Q'*dq;omega2(4)=0;
        dq=Q*omega2;
    
        y(qindex2(:,i))=q;
        y(qindex(:,i))=dq;
        
    end
    

end

== matlab function DQ_SR_LIB_SIM/DQ Kinematics fixed mass/MATLAB Function2 ==
  data: t input; dy output; DCG output size=6; state input size=[n_var,1]; CG input size=6; II parameter; ext_f input size=[n_ext]; sys_gen_fun_NAME parameter; gravity_fun_NAME parameter
function [dy,DCG] = DQ_coreCM(t,state,CG,II,ext_f,sys_gen_fun_NAME,gravity_fun_NAME)
%#codegen


% cg variables
vcg=CG(1:3);
xcg=CG(4:6);


% user defined functions
sys_gen_fun=str2func(char(sys_gen_fun_NAME));
gravity_fun=str2func(char(gravity_fun_NAME));


% system computation
[ddx]=dynamicsCM(t,state,xcg,vcg,II,ext_f,sys_gen_fun,gravity_fun);

n_var=length(state)/2;

% outputs
dy=[ddx(1:(n_var),1);ddx((n_var+4):end-3,1)];
DCG=[ddx(n_var+1:n_var+3,1);ddx((end-2):end,1)];

== matlab function DQ_SR_LIB_SIM/Utilities/Body angular velocity/MATLAB Function ==
  data: q input; omega output; dq input
function omega = fcn(q,dq)
%#codegen


QPT=crossqp(q)';
QPT=QPT(1:3,:);
omega=2*QPT*dq;

== matlab function DQ_SR_LIB_SIM/DQ Kinematics Ground fixed mass/MATLAB Function ==
  data: u input; x output; dx output; n_states parameter
function [x,dx] = fcn(u,n_states)
%#codegen

% velocity and position of cg included

dx = u (1:(n_states/2),1);

x = u ((n_states/2+1):n_states,1);

== matlab function DQ_SR_LIB_SIM/DQ Kinematics Ground fixed mass/MATLAB Function1 ==
  data: u input; y output; index parameter; index2 parameter
function y = quatnormalize(u,index,index2)
%#codegen


q=u(index);
dq=u(index2);

% quat norm
q=q./norm(q);

% dquat norm
Q=crossqm(q);
omega2=Q'*dq;omega2(4)=0;
dq=Q*omega2;




y = u;
y(index)=q;
y(index2)=dq;

== matlab function DQ_SR_LIB_SIM/DQ Kinematics Ground fixed mass/MATLAB Function2 ==
  data: t input; dy output; a output; da output; dda output; state input size=[n_var,1]; II parameter; ext_f input size=[n_ext]; sys_gen_fun_NAME parameter; gravity_fun_NAME parameter; n_bodies parameter size=1
function [dy,a,da,dda] = DQ_core(t,state,II,ext_f,sys_gen_fun_NAME,gravity_fun_NAME,n_bodies)
%#codegen


% user defined functions
sys_gen_fun=str2func(char(sys_gen_fun_NAME));
gravity_fun=str2func(char(gravity_fun_NAME));


% system computation
[ddx,a,da,dda]=dynamicsG(t,state,II,ext_f,sys_gen_fun,gravity_fun,n_bodies);

n_var=length(state)/2;

% outputs
dy=[ddx(1:(n_var),1);ddx((n_var+4):end-3,1)];
DCG=[ddx(n_var+1:n_var+3,1);ddx((end-2):end,1)];

== matlab function DQ_SR_LIB_SIM/DQ Kinematics fixed mass/MATLAB Function3 ==
  data: t input; state input size=[n_var,1]; a output; CG input size=6; II parameter; n_ext parameter; sys_gen_fun_NAME parameter; n_bodies parameter size=1; da output
function [a,da] = get_the_dq_state(t,state,CG,II,n_ext,sys_gen_fun_NAME,n_bodies)
%#codegen


% cg variables
vcg=CG(1:3);
xcg=CG(4:6);

% state dimension
n_var=length(state)/2;

% get state and its derivative
dx=state(1:n_var);
x=state(n_var+1:end);




% user defined functions
sys_gen_fun=str2func(char(sys_gen_fun_NAME));



% extract all the states
[SYS]=sys_gen_fun(x,dx,xcg,vcg,t,II,zeros(n_ext,1),[],[]);

% enforce the constraints
SYS=enforce_cg_constr(SYS);

% % extract the state 
[a,da]=getfullstate(SYS,n_bodies);

== matlab function DQ_SR_LIB_SIM/DQ Kinematics Variable mass/MATLAB Function2 ==
  data: t input; dy output; DCG output size=6; dxi output size=[n_massvar]; state input size=[n_var,1]; CG input size=6; xi input size=[n_massvar]; II parameter; ext_f input size=[n_ext]; sys_gen_fun_NAME parameter; gravity_fun_NAME parameter
function [dy,DCG,dxi] = DQ_coreVM(t,state,CG,xi,II,ext_f,sys_gen_fun_NAME,gravity_fun_NAME)
%#codegen


% cg variables
vcg=CG(1:3);
xcg=CG(4:6);


% user defined functions
sys_gen_fun=str2func(char(sys_gen_fun_NAME));
gravity_fun=str2func(char(gravity_fun_NAME));


% system computation
[ddx,dxi]=dynamicsVM(t,state,xcg,vcg,xi,II,ext_f,sys_gen_fun,gravity_fun);

n_var=length(state)/2;

% outputs
dy=[ddx(1:(n_var),1);ddx((n_var+4):end-3,1)];
DCG=[ddx(n_var+1:n_var+3,1);ddx((end-2):end,1)];

== matlab function DQ_SR_LIB_SIM/DQ Kinematics Variable mass/MATLAB Function3 ==
  data: t input; state input size=[n_var,1]; a output; CG input size=6; xi input; II parameter; n_ext parameter; sys_gen_fun_NAME parameter; n_bodies parameter size=1; da output
function [a,da] = get_the_dq_stateVM(t,state,CG,xi,II,n_ext,sys_gen_fun_NAME,n_bodies)
%#codegen


% cg variables
vcg=CG(1:3);
xcg=CG(4:6);

% state dimension
n_var=length(state)/2;

% get state and its derivative
dx=state(1:n_var);
x=state(n_var+1:end);




% user defined functions
sys_gen_fun=str2func(char(sys_gen_fun_NAME));



% extract all the states
[SYS]=sys_gen_fun(x,dx,xcg,vcg,t,II,zeros(n_ext,1),xi,[]);

% enforce the constraints
SYS=enforce_cg_constr(SYS);

% extract the state 
[a,da]=getfullstate(SYS,n_bodies);

== matlab function DQ_SR_LIB_SIM/Utilities/Inertial angular velocity/MATLAB Function ==
  data: q input; omega output; dq input
function omega = fcn(q,dq)
%#codegen


QMT=crossqm(q)';
QMT=QMT(1:3,:);
omega=2*QMT*dq;

== matlab function DQ_SR_LIB_SIM/Utilities/Inertial position/MATLAB Function ==
  data: a input size=[8,1]; d output size=[3,1]
function d = fcn(a)
%#codegen


QMT=crossqm(a(1:4))';
QMT=QMT(1:3,:);
d=2*QMT*a(5:8);

== matlab function DQ_SR_LIB_SIM/Utilities/Body position/MATLAB Function ==
  data: a input; d output
function d = fcn(a)
%#codegen


QPT=crossqp(a(1:4))';
QPT=QPT(1:3,:);
d=2*QPT*a(5:8);

== matlab function DQ_SR_LIB_SIM/DQ Kinematics fixed mass multiple systems/MATLAB Function ==
  data: u input; x output; dx output; n_states parameter
function [x,dx] = fcn(u,n_states)
%#codegen

% velocity and position of cg included

dx = u (1:(n_states/2),1);

x = u ((n_states/2+1):n_states,1);

== matlab function DQ_SR_LIB_SIM/DQ Kinematics fixed mass multiple systems/MATLAB Function4 ==
  data: u input; y output; qindex parameter; NORMONOFF parameter
function y = quatnormalize(u,qindex,NORMONOFF)
%#codegen

y = u;

if NORMONOFF

    n_state=length(u)/2; % number of states
    
    qindex2=qindex+(n_state); %get quaternion index
    
    
    for i=1:size(qindex,2)
    
        % extract quaternion and its derivative
        q=u(qindex2(:,i));
        dq=u(qindex(:,i));
        
        % quat norm
        q=q./norm(q);
        
        % dquat norm
        Q=crossqm(q);
        omega2=Q'*dq;omega2(4)=0;
        dq=Q*omega2;
    
        y(qindex2(:,i))=q;
        y(qindex(:,i))=dq;
        
    end
    

end
